simulink model "testmodels"  (Simulink 7.6)
settings: Solver=ode45  StartTime=0.0  StopTime=10.0  RelTol=1e-3
undefined symbols (not defined in the file or in its folder): vec1
settings Model: Creator=root  LastModifiedBy=root

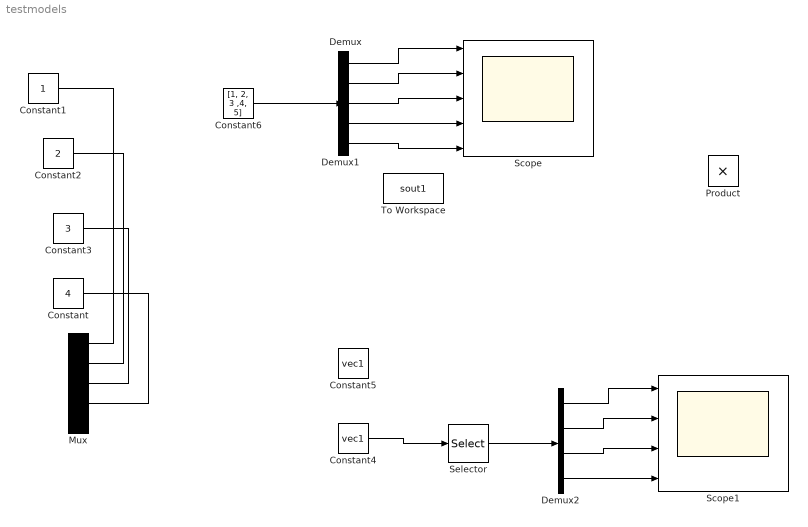
== system testmodels ==
  Constant : Constant  Value=4
  Constant1 : Constant
  Constant2 : Constant  Value=2
  Constant3 : Constant  Value=3
  Constant4 : Constant  Value=vec1  VectorParams1D=off
  Constant5 : Constant  Value=vec1  VectorParams1D=off
  Constant6 : Constant  Value=[1, 2, 3 ,4, 5]
  Demux : Demux  Outputs=5
  Demux1 : Demux  Outputs=5
  Demux2 : Demux
  Mux : Mux  Inputs=5
  Product : Product  RndMeth=Zero
  Scope : Scope  NumInputPorts=5
      settings: YMin=-5~-5~-5~-5~-5  YMax=5~5~5~5~5
  Scope1 : Scope  NumInputPorts=4
      settings: YMin=-5~-5~-5~-5  YMax=5~5~5~5
  Selector : Selector  InputPortWidth=5  IndexOptions=Starting index (dialog)  Indices=2  OutputSizes=4
  To Workspace : ToWorkspace  VariableName=sout1  SampleTime=-1  SaveFormat=Array
  wires:
  Demux/1 -> Scope/1
  Demux/2 -> Scope/2
  Demux/3 -> Scope/3
  Demux/4 -> Scope/4
  Demux/5 -> Scope/5
  Constant1/1 -> Mux/1
  Constant2/1 -> Mux/2
  Constant3/1 -> Mux/3
  Constant/1 -> Mux/4
  Constant4/1 -> Selector/1
  Selector/1 -> Demux2/1
  Demux2/1 -> Scope1/1
  Demux2/2 -> Scope1/2
  Demux2/3 -> Scope1/3
  Demux2/4 -> Scope1/4
  Constant6/1 -> Demux/1
